simulink model "testtest22"  (Simulink 7.6)
settings: Solver=ode45  StartTime=0.0  StopTime=2000  RelTol=1e-3
values from neighbouring files (symbols this model uses):
  K = [9.375  -6.25; -8.125  8.75]    [PP2013428.mat]
libraries: ADRC x2
settings Model: Creator=Administrator  LastModifiedBy=Administrator
settings DebuggingCC: AlgebraicLoopMsg=none  ArtificialAlgebraicLoopMsg=none  SolverPrmCheckMsg=none  UnknownTsInhSupMsg=none

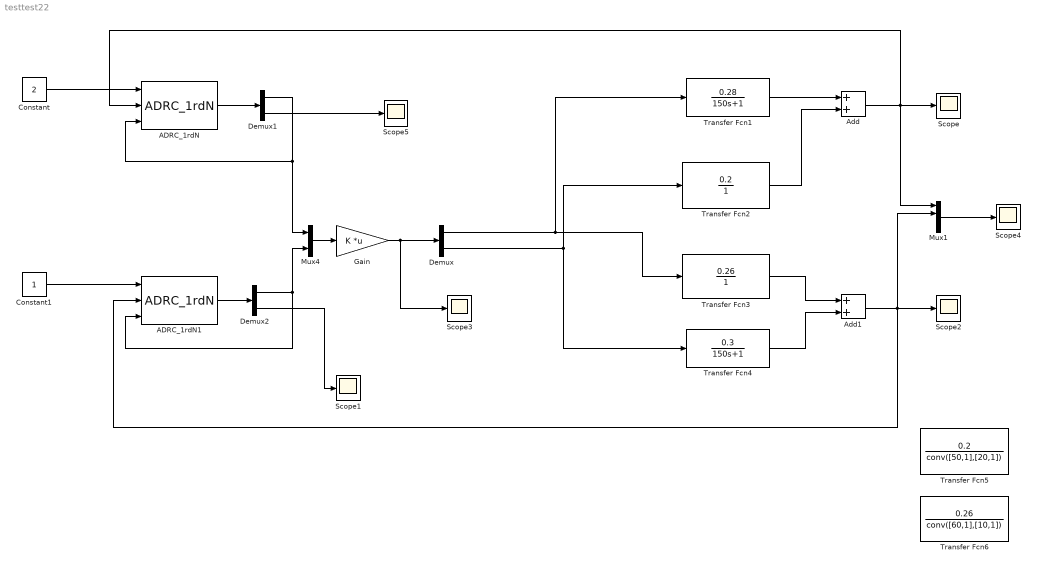
== system testtest22 ==
  ADRC_1rdN : ADRC/ADRC/ADRC_1rd/ADRC_1rdN  SystemSampleTime=-1  RT=50  h=0.05  B01=20  B02=80  r=1
  ADRC_1rdN1 : ADRC/ADRC/ADRC_1rd/ADRC_1rdN  SystemSampleTime=-1  RT=400  h=0.05  B01=20  B02=80  r=1
  Add : Sum
  Add1 : Sum
  Constant : Constant  Value=2
  Constant1 : Constant
  Demux : Demux  Outputs=2
  Demux1 : Demux  Outputs=2
  Demux2 : Demux  Outputs=2
  Gain : Gain  Gain=K  Multiplication=Matrix(K*u)
  Mux1 : Mux
  Mux4 : Mux  Inputs=2
  Scope{,1..5} (6 alike) : Scope
      Scope settings: TimeRange=1000  YMin=-2e+235  YMax=1.4e+236  DataFormat=Array
      Scope1 settings: TimeRange=1000  YMin=-2e+235  YMax=1.4e+236  SaveName=ScopeData4  DataFormat=Array
      Scope2 settings: YMin=5.25  YMax=10.25  SaveName=ScopeData2  DataFormat=Array
      Scope3 settings: TimeRange=1000  YMin=-2e+235  YMax=1.4e+236  SaveName=ScopeData3  DataFormat=Array
      Scope4 settings: TimeRange=2000  YMin=1  YMax=6.75  DataFormat=Array
      Scope5 settings: TimeRange=1000  YMin=-2e+235  YMax=1.4e+236  SaveName=ScopeData5  DataFormat=Array
  Transfer Fcn1 : TransferFcn  Numerator=0.28  Denominator=[150 1]
  Transfer Fcn2 : TransferFcn  Numerator=0.2  Denominator=1
  Transfer Fcn3 : TransferFcn  Numerator=0.26  Denominator=1
  Transfer Fcn4 : TransferFcn  Numerator=0.3  Denominator=[150,1]
  Transfer Fcn5 : TransferFcn  Numerator=0.2  Denominator=conv([50,1],[20,1])
  Transfer Fcn6 : TransferFcn  Numerator=0.26  Denominator=conv([60,1],[10,1])
  wires:
  Transfer Fcn3/1 -> Add1/1
  Transfer Fcn4/1 -> Add1/2
  Add1/1 -> Scope2/1, ADRC_1rdN1/2, Mux1/2
  Constant1/1 -> ADRC_1rdN1/1
  ADRC_1rdN1/1 -> Demux2/1
  Demux2/1 -> ADRC_1rdN1/3, Mux4/2
  Demux/2 -> Transfer Fcn4/1, Transfer Fcn2/1
  Constant/1 -> ADRC_1rdN/1
  ADRC_1rdN/1 -> Demux1/1
  Mux4/1 -> Gain/1
  Gain/1 -> Demux/1, Scope3/1
  Demux/1 -> Transfer Fcn1/1, Transfer Fcn3/1
  Transfer Fcn1/1 -> Add/1
  Transfer Fcn2/1 -> Add/2
  Add/1 -> Scope/1, ADRC_1rdN/2, Mux1/1
  Demux1/1 -> Mux4/1, ADRC_1rdN/3
  Mux1/1 -> Scope4/1
  Demux2/2 -> Scope1/1
  Demux1/2 -> Scope5/1
